simulink model "Hardware_Code"  (R2025b)
settings: Solver=FixedStepAuto  StartTime=0.0  StopTime=30  RelTol=1e-3  EnableMultiTasking=on
InitFcn:
  | battery_init;
  | Full_Charge_Volt=4.2; % unit volts
  | Cutoff_Volt=3; % unit volts
  | Delta=.02;
  | ContactorTime=20;
  | ContactorTimeOut=100;
  | High_TempLim=333;
  | Low_TempLim=253;
  | Sensor_Fault_Treshold=.02;
  | CurrentTimeout=1;
  | Allowed_Delta=.04;
  | Bal_On_Time=30;
  | Bal_Off_Time=5;
  | BalNotAct_Time=10;
values from neighbouring files (symbols this model uses):
  Charge_Rate = 1    [battery_init.m]
  Discharge_Rate = -1    [battery_init.m]
  Fly_Cycle_Current = [ ... (first row only)    [battery_init.m]
undefined symbols (not defined in the file or in its folder): batt, From_Plant_MATLABStruct, SRE
libraries: fl_lib x69, nesl_utility x54, ee_lib x12, batteryecm_lib x12, simulink x6, BatteryCurrentManagement x1
(part 2 of 2)

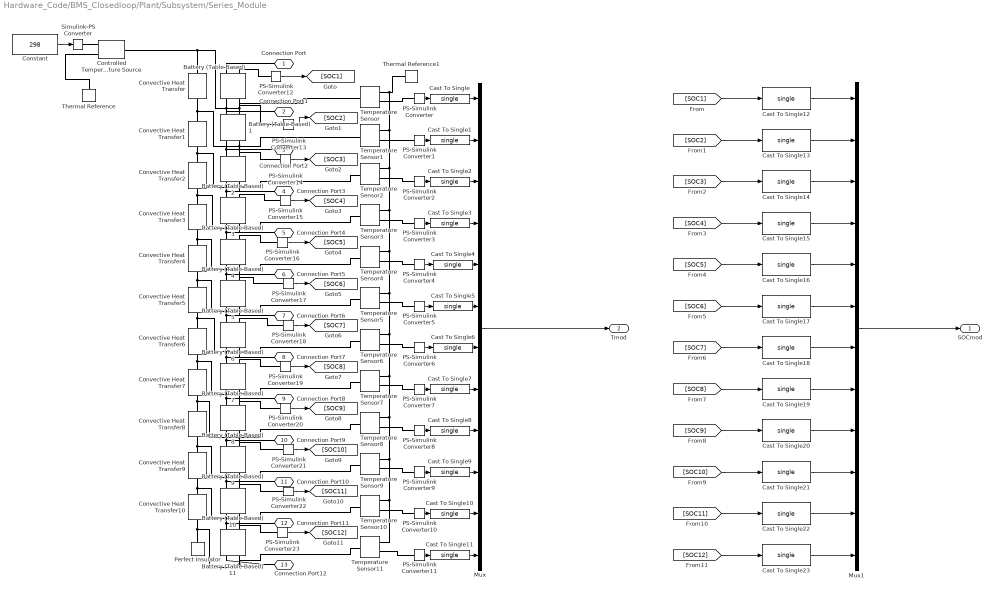
== system Hardware_Code/BMS_Closedloop/Plant/Subsystem/Series_Module ==
  Battery (Table-Based){,1..11} (12 alike) : batteryecm_lib/Battery (Table-Based)  PartSpecification="{\"CollectionId\":\"SimscapeBatteryShared\",\"CollectionVersion\":\"1.0.0\",\"DatasetId\":\"Molicel|INR_21700_P45B|simscape.battery.batteryTableBased\",\"DisplayName\":\"Molicel:INR_21700_P45B\"}"  SOC_vec=[0 0.01 0.02 0.03 0.04 0.05 0.06 0.07 0.08 0.09 0.1 0.11 0.12 0.13 0.14 0.15 0.16 0.17 0.18 0.19 0.2 0.21 0.22 0.23 0.24 0.25 0.26 0.27 0.28 0.29 0.3 0.31 0.32 0.33 0.34 0.35 0.36 0.37 0.38 0.39 0.4 0.41 0.42 0.43 0.44 0.45 0.46 0.47 0.48 0.49 0.5 0.51 0.52 0.53 0.54 0.55 0.56 0.57 0.58 0.59 0.6 0.61 0.62 0.63 0.64 0.65 0.66 0.67 0.68 0.69 0.7 0.71 0.72 0.73 0.74 0.75 0.76 0.77 0.78 0.79 0.8 0.81 0.82 0.83 0.84 0.85 0.86 0.87 0.88 0.89 0.9 0.91 0.92 0.93 0.94 0.95 0.96 0.97 0.98 0.99 1] % Datasheet derived  T_dependence=simscape.enum.tablebattery.temperature_dependence.yes  prm_dir=simscape.enum.tablebattery.prm_dir.noCurrentDirectionality  T_vec=[233.15 243.15 253.15 273.15 296.15 318.15 333.15] K  V0_mat=[3.17242 3.17242 3.17242 3.17242 3.17242 3.17242 3.17242;3.18272 3.18272 3.18272 3.18272 3.18272 3.18272 3.18272;3.19302 3.19302 3.19302 3.19302 3.19302 3.19302 3.19302;3.20331 3.20331 3.20331 3.20331 3.20331 3.20331 3.20331;3.21361 3.21361 3.21361 3.21361 3.21361 3.21361 3.21361;3.22391 3.22391 3.22391 3.22391 3.22391 3.22391 3.22391;3.23421 3.23421 3.23421 3.23421 3.23421 3.23421 3.23421;3.24451 3.24451 3.24451 3.24451 3.24451 3.24451 3.24451;3.25481 3.25481 3.25481 3.25481 3.25481 3.25481 3.25481;3.2651 3.2651 3.2651 3.2651 3.2651 3.2651 3.2651;3.2754 3.2754 3.2754 3.2754 3.2754 3.2754 3.2754;3.2857 3.2857 3.2857 3.2857 3.2857 3.2857 3.2857;3.296 3.296 3.296 3.296 3.296 3.296 3.296;3.3063 3.3063 3.3063 3.3063 3.3063 3.3063 3.3063;3.31659 3.31659 3.31659 3.31659 3.31659 3.31659 3.31659;3.32689 3.32689 3.32689 3.32689 3.32689 3.32689 3.32689;3.33719 3.33719 3.33719 3.33719 3.33719 3.33719 3.33719;3.34749 3.34749 3.34749 3.34749 3.34749 3.34749 3.34749;3.35779 3.35779 3.35779 3.35779 3.35779 3.35779 3.35779;3.36809 3.36809 3.36809 3.36809 3.36809 3.36809 3.36809;3.37838 3.37838 3.37838 3.37838 3.37838 3.37838 3.37838;3.38868 3.38868 3.38868 3.38868 3.38868 3.38868 3.38868;3.39898 3.39898 3.39898 3.39898 3.39898 3.39898 3.39898;3.40928 3.40928 3.40928 3.40928 3.40928 3.40928 3.40928;3.41958 3.41958 3.41958 3.41958 3.41958 3.41958 3.41958;3.42988 3.42988 3.42988 3.42988 3.42988 3.42988 3.42988;3.44017 3.44017 3.44017 3.44017 3.44017 3.44017 3.44017;3.45047 3.45047 3.45047 3.45047 3.45047 3.45047 3.45047;3.46077 3.46077 3.46077 3.46077 3.46077 3.46077 3.46077;3.47107 3.47107 3.47107 3.47107 3.47107 3.47107 3.47107;3.48137 3.48137 3.48137 3.48137 3.48137 3.48137 3.48137;3.49166 3.49166 3.49166 3.49166 3.49166 3.49166 3.49166;3.50196 3.50196 3.50196 3.50196 3.50196 3.50196 3.50196;3.51226 3.51226 3.51226 3.51226 3.51226 3.51226 3.51226;3.52256 3.52256 3.52256 3.52256 3.52256 3.52256 3.52256;3.53286 3.53286 3.53286 3.53286 3.53286 3.53286 3.53286;3.54316 3.54316 3.54316 3.54316 3.54316 3.54316 3.54316;3.55345 3.55345 3.55345 3.55345 3.55345 3.55345 3.55345;3.56375 3.56375 3.56375 3.56375 3.56375 3.56375 3.56375;3.57405 3.57405 3.57405 3.57405 3.57405 3.57405 3.57405;3.58435 3.58435 3.58435 3.58435 3.58435 3.58435 3.58435;3.59465 3.59465 3.59465 3.59465 3.59465 3.59465 3.59465;3.60495 3.60495 3.60495 3.60495 3.60495 3.60495 3.60495;3.61524 3.61524 3.61524 3.61524 3.61524 3.61524 3.61524;3.62554 3.62554 3.62554 3.62554 3.62554 3.62554 3.62554;3.63584 3.63584 3.63584 3.63584 3.63584 3.63584 3.63584;3.64614 3.64614 3.64614 3.64614 3.64614 3.64614 3.64614;3.65644 3.65644 3.65644 3.65644 3.65644 3.65644 3.65644;3.66673 3.66673 3.66673 3.66673 3.66673 3.66673 3.66673;3.67703 3.67703 3.67703 3.67703 3.67703 3.67703 3.67703;3.68733 3.68733 3.68733 3.68733 3.68733 3.68733 3.68733;3.69763 3.69763 3.69763 3.69763 3.69763 3.69763 3.69763;3.71041 3.71041 3.71041 3.71041 3.71041 3.71041 3.71041;3.72113 3.72113 3.72113 3.72113 3.72113 3.72113 3.72113;3.72997 3.72997 3.72997 3.72997 3.72997 3.72997 3.72997;3.73882 3.73882 3.73882 3.73882 3.73882 3.73882 3.73882;3.74912 3.74912 3.74912 3.74912 3.74912 3.74912 3.74912;3.75936 3.75936 3.75936 3.75936 3.75936 3.75936 3.75936;3.76951 3.76951 3.76951 3.76951 3.76951 3.76951 3.76951;3.7791 3.7791 3.7791 3.7791 3.7791 3.7791 3.7791;3.78865 3.78865 3.78865 3.78865 3.78865 3.78865 3.78865;3.79787 3.79787 3.79787 3.79787 3.79787 3.79787 3.79787;3.80709 3.80709 3.80709 3.80709 3.80709 3.80709 3.80709;3.8161 3.8161 3.8161 3.8161 3.8161 3.8161 3.8161;3.82509 3.82509 3.82509 3.82509 3.82509 3.82509 3.82509;3.83409 3.83409 3.83409 3.83409 3.83409 3.83409 3.83409;3.84308 3.84308 3.84308 3.84308 3.84308 3.84308 3.84308;3.85207 3.85207 3.85207 3.85207 3.85207 3.85207 3.85207;3.86107 3.86107 3.86107 3.86107 3.86107 3.86107 3.86107;3.87006 3.87006 3.87006 3.87006 3.87006 3.87006 3.87006;3.87901 3.87901 3.87901 3.87901 3.87901 3.87901 3.87901;3.88831 3.88831 3.88831 3.88831 3.88831 3.88831 3.88831;3.89824 3.89824 ...(+1594 chars)] % Datasheet derived V  V0_vec=[3.17242 3.18272 3.19302 3.20331 3.21361 3.22391 3.23421 3.24451 3.25481 3.2651 3.2754 3.2857 3.296 3.3063 3.31659 3.32689 3.33719 3.34749 3.35779 3.36809 3.37838 3.38868 3.39898 3.40928 3.41958 3.42988 3.44017 3.45047 3.46077 3.47107 3.48137 3.49166 3.50196 3.51226 3.52256 3.53286 3.54316 3.55345 3.56375 3.57405 3.58435 3.59465 3.60495 3.61524 3.62554 3.63584 3.64614 3.65644 3.66673 3.67703 3.68733 3.69763 3.71041 3.72113 3.72997 3.73882 3.74912 3.75936 3.76951 3.7791 3.78865 3.79787 3.80709 3.8161 3.82509 3.83409 3.84308 3.85207 3.86107 3.87006 3.87901 3.88831 3.89824 3.90887 3.91951 3.93012 3.94073 3.95138 3.96184 3.97226 3.98268 3.99311 4.0032 4.01221 4.01944 4.02668 4.03286 4.03874 4.04383 4.0488 4.05377 4.05873 4.06312 4.06753 4.07333 4.08117 4.08904 4.09911 4.11111 4.13802 4.16831] % Datasheet derived V  V_range=[2.25 Inf] % Datasheet derived V  R0_mat=[0.3026 0.35142 0.34349 0.24415 0.02095 0.15874 0.14729;0.2941 0.33555 0.32379 0.22614 0.01921 0.13363 0.12249;0.28559 0.31969 0.30408 0.20813 0.01774 0.10853 0.10276;0.27709 0.30382 0.28438 0.19012 0.0166 0.09423 0.0861;0.26858 0.28796 0.26468 0.17211 0.01557 0.07998 0.0748;0.26008 0.27209 0.24498 0.1541 0.01469 0.07024 0.06679;0.25157 0.25623 0.22527 0.1361 0.01398 0.06387 0.05877;0.24307 0.24036 0.20557 0.11861 0.01338 0.0575 0.05275;0.23456 0.2245 0.18587 0.10674 0.01283 0.05113 0.04899;0.22606 0.20863 0.16617 0.09525 0.01239 0.04679 0.04522;0.21755 0.19277 0.14651 0.08799 0.01196 0.0439 0.04145;0.20905 0.1769 0.13098 0.08073 0.01155 0.04101 0.03817;0.20054 0.16103 0.11905 0.07347 0.01116 0.03813 0.03522;0.19204 0.14769 0.11102 0.06895 0.01079 0.03524 0.03228;0.18353 0.13913 0.10517 0.06499 0.01042 0.03235 0.02934;0.17503 0.13157 0.09933 0.06104 0.01007 0.02946 0.0264;0.16653 0.1271 0.09371 0.05708 0.00974 0.02657 0.02345;0.15804 0.12264 0.09094 0.05312 0.00949 0.02417 0.02125;0.15354 0.11817 0.08816 0.04917 0.00924 0.02286 0.01972;0.14976 0.11385 0.08539 0.04748 0.009 0.02156 0.0182;0.14598 0.11213 0.08261 0.04617 0.00876 0.02025 0.01667;0.14219 0.11042 0.08103 0.04487 0.00855 0.01894 0.01515;0.14033 0.10871 0.08035 0.04356 0.00843 0.01763 0.01363;0.13876 0.10699 0.07967 0.04225 0.00832 0.01632 0.0121;0.13718 0.10528 0.07899 0.04094 0.00826 0.01501 0.01058;0.13561 0.10357 0.07831 0.03964 0.00825 0.0137 0.00906;0.13404 0.10198 0.07763 0.03833 0.00825 0.01239 0.00753;0.13247 0.10119 0.07695 0.03702 0.00826 0.01108 0.0065;0.13096 0.10039 0.07627 0.03624 0.00827 0.00977 0.00633;0.13043 0.0996 0.07559 0.03615 0.00828 0.00846 0.00617;0.1299 0.0988 0.07491 0.03606 0.0083 0.00774 0.006;0.12937 0.09801 0.07423 0.03597 0.00834 0.00779 0.00583;0.12883 0.09721 0.07355 0.03588 0.00838 0.00783 0.00567;0.1283 0.09642 0.07301 0.03579 0.00842 0.00787 0.0055;0.12777 0.09585 0.07296 0.0357 0.00848 0.00792 0.00534;0.12724 0.09584 0.07291 0.03561 0.00855 0.00796 0.00517;0.12675 0.09584 0.07286 0.03552 0.00863 0.00801 0.005;0.12643 0.09583 0.0728 0.03543 0.00871 0.00805 0.00484;0.12611 0.09582 0.07275 0.03534 0.00879 0.00809 0.00467;0.12579 0.09582 0.0727 0.03525 0.00887 0.00814 0.0045;0.12547 0.09581 0.07264 0.03526 0.00895 0.00818 0.00434;0.12514 0.0958 0.07259 0.03537 0.00903 0.00823 0.00405;0.12482 0.09579 0.07254 0.03547 0.00911 0.00804 0.00366;0.1245 0.09579 0.07248 0.03558 0.00918 0.00776 0.00327;0.12418 0.09578 0.07243 0.03568 0.00925 0.00748 0.00287;0.12386 0.09577 0.07231 0.03579 0.00931 0.0072 0.00248;0.12354 0.09576 0.0721 0.03589 0.00938 0.00692 0.00209;0.12322 0.09576 0.07189 0.036 0.00946 0.00664 0.0017;0.12301 0.09575 0.07168 0.03611 0.00953 0.00636 0.00131;0.12309 0.09574 0.07147 0.03621 0.00961 0.00608 0.00092;0.12318 0.09573 0.07125 0.0363 0.00968 0.0058 0.00053;0.12326 0.09573 0.07104 0.03637 0.00976 0.00552 0.00014;0.12389 0.09628 0.07138 0.03699 0.00991 0.00579 0.0003;0.12407 0.09637 0.07126 0.03715 0.01 0.0056 0.0003;0.12383 0.09605 0.07073 0.0369 0.01003 0.00504 0.0003;0.12359 0.09573 0.07019 0.03664 0.01006 0.00503 0.0003;0.12367 0.09573 0.06998 0.03671 0.01013 0.00534 0.00063;0.12375 0.09572 0.06975 0.03677 0.01022 0.00564 0.00094;0.1238 0.09569 0.07006 0.0368 0.0103 0.00593 0.00123;0.12372 0.09554 0.07026 0.03671 0.01037 0.00608 0.00139;0.12364 0.09537 0.07046 0.03661 0.01043 0.00623 0.00155;0.12348 0.09514 0.07058 0.03644 0.01049 0.0063 0.00163;0.12333 0.0949 0.07071 0.03627 0.01055 0.00638 0.00171;0.12312 0.09461 0.07078 0.03605 0.01061 0.00641 0.00175;0.12291 0.09433 0.07085 0.03583 0.01066 0.00643 0.00168;0.12271 0.09404 0.07093 0.03568 0.01072 0.00646 0.00161;0.12275 0.09398 0.071 0.03622 0.01077 0.00646 0.00153;0.12316 0.09449 0.07107 0.03677 0.01082 0.00636 0.00145;0.12357 0.095 0.07115 0.03731 0.01088 0.00625 0.00137;0.12398 0.09551 0.07151 0.03785 0.01093 0.00614 0.00129;0.12438 0.09601 0.07221 0.03839 0.01099 0.00602 0.0012;0.12486 0.09659 0.07299 0.039 0.01105 0.00599 0.00119;0.12548 0.09731 0.07391 ...(+1579 chars)] % Datasheet derived Ohm  R0_vec=[0.02095 0.01921 0.01774 0.0166 0.01557 0.01469 0.01398 0.01338 0.01283 0.01239 0.01196 0.01155 0.01116 0.01079 0.01042 0.01007 0.00974 0.00949 0.00924 0.009 0.00876 0.00855 0.00843 0.00832 0.00826 0.00825 0.00825 0.00826 0.00827 0.00828 0.0083 0.00834 0.00838 0.00842 0.00848 0.00855 0.00863 0.00871 0.00879 0.00887 0.00895 0.00903 0.00911 0.00918 0.00925 0.00931 0.00938 0.00946 0.00953 0.00961 0.00968 0.00976 0.00991 0.01 0.01003 0.01006 0.01013 0.01022 0.0103 0.01037 0.01043 0.01049 0.01055 0.01061 0.01066 0.01072 0.01077 0.01082 0.01088 0.01093 0.01099 0.01105 0.01114 0.01125 0.01136 0.01148 0.01161 0.01175 0.01188 0.01202 0.01215 0.01228 0.01241 0.01253 0.01261 0.01269 0.01275 0.0128 0.01285 0.01289 0.01294 0.01298 0.01296 0.01292 0.01292 0.01288 0.01282 0.0128 0.01232 0.01214 0.00952] % Datasheet derived Ohm  R0_dis_mat=[.0117, .0085, .009; .011, .0085, .009; .0114, .0087, .0092; .0107, .0082, .0088; .0107, .0083, .0091; .0113, .0085, .0089; .0116, .0085, .0089] % Parameter not set Ohm  R0_dis_vec=[.0085, .0085, .0087, .0082, .0083, .0085, .0085] % Parameter not set Ohm  R0_ch_mat=[.0117, .0085, .009; .011, .0085, .009; .0114, .0087, .0092; .0107, .0082, .0088; .0107, .0083, .0091; .0113, .0085, .0089; .0116, .0085, .0089] % Parameter not set Ohm  R0_ch_vec=[.0085, .0085, .0087, .0082, .0083, .0085, .0085] % Parameter not set Ohm  AH=4.493 % Datasheet derived hr*A  prm_leak=simscape.enum.tablebattery.prm_leak.disabled  Rleak_vec=[8000, 7000, 6000] % Parameter not set Ohm  Rleak=7e3 % Parameter not set Ohm  extrapolation_option=simscape.enum.extrapolation.nearest  SOC_port=simscape.enum.tablebattery.enable.yes  prm_dyn=simscape.enum.tablebattery.prm_dyn.off  R1_mat=[.0109, .0029, .0013; .0069, .0024, .0012; .0047, .0026, .0013; .0034, .0016, .001; .0033, .0023, .0014; .0033, .0018, .0011; .0028, .0017, .0011] % Parameter not set Ohm  R1_vec=[.0029, .0024, .0026, .0016, .0023, .0018, .0017] % Parameter not set Ohm  tau1_mat=[20, 36, 39; 31, 45, 39; 109, 105, 61; 36, 29, 26; 59, 77, 67; 40, 33, 29; 25, 39, 33] % Parameter not set s  tau1_vec=[36, 45, 105, 29, 77, 33, 39] % Parameter not set s  R2_mat=[.0109, .0029, .0013; .0069, .0024, .0012; .0047, .0026, .0013; .0034, .0016, .001; .0033, .0023, .0014; .0033, .0018, .0011; .0028, .0017, .0011] % Parameter not set Ohm  R2_vec=[.0029, .0024, .0026, .0016, .0023, .0018, .0017] % Parameter not set Ohm  tau2_mat=[20, 36, 39; 31, 45, 39; 109, 105, 61; 36, 29, 26; 59, 77, 67; 40, 33, 29; 25, 39, 33] % Parameter not set s  tau2_vec=[36, 45, 105, 29, 77, 33, 39] % Parameter not set s  R3_mat=[.0109, .0029, .0013; .0069, .0024, .0012; .0047, .0026, .0013; .0034, .0016, .001; .0033, .0023, .0014; .0033, .0018, .0011; .0028, .0017, .0011] % Parameter not set Ohm  R3_vec=[.0029, .0024, .0026, .0016, .0023, .0018, .0017] % Parameter not set Ohm  tau3_mat=[20, 36, 39; 31, 45, 39; 109, 105, 61; 36, 29, 26; 59, 77, 67; 40, 33, 29; 25, 39, 33] % Parameter not set s  tau3_vec=[36, 45, 105, 29, 77, 33, 39] % Parameter not set s  R4_mat=[.0109, .0029, .0013; .0069, .0024, .0012; .0047, .0026, .0013; .0034, .0016, .001; .0033, .0023, .0014; .0033, .0018, .0011; .0028, .0017, .0011] % Parameter not set Ohm  R4_vec=[.0029, .0024, .0026, .0016, .0023, .0018, .0017] % Parameter not set Ohm  tau4_mat=[20, 36, 39; 31, 45, 39; 109, 105, 61; 36, 29, 26; 59, 77, 67; 40, 33, 29; 25, 39, 33] % Parameter not set s  tau4_vec=[36, 45, 105, 29, 77, 33, 39] % Parameter not set s  R5_mat=[.0109, .0029, .0013; .0069, .0024, .0012; .0047, .0026, .0013; .0034, .0016, .001; .0033, .0023, .0014; .0033, .0018, .0011; .0028, .0017, .0011] % Parameter not set Ohm  R5_vec=[.0029, .0024, .0026, .0016, .0023, .0018, .0017] % Parameter not set Ohm  tau5_mat=[20, 36, 39; 31, 45, 39; 109, 105, 61; 36, 29, 26; 59, 77, 67; 40, 33, 29; 25, 39, 33] % Parameter not set s  tau5_vec=[36, 45, 105, 29, 77, 33, 39] % Parameter not set s  prm_fade=simscape.enum.tablebattery.prm_fade.tableN  N0=100 % Parameter not set  dV0=0 % Parameter not set  dR0=0 % Parameter not set  dAH=0 % Parameter not set  dRleak=0 % Parameter not set  dR1=0 % Parameter not set  dR2=0 % Parameter not set  dR3=0 % Parameter not set  dR4=0 % Parameter not set  dR5=0 % Parameter not set  N0vec=[0 6 11 16 21 26 31 36 41 46 51 56 61 66 71 76 81 86 91 96 101 106 111 116 121 126 131 136 141 146 151 156 161 166 171 176 181 186 191 196 201 206 211 216 221 226 231 236 241 246 251 256 261 266 271 276 281 286 291 296 301 306 311 316 321 326 331 336 341 346 351 356 361 366 371 376 381 386 391 396 401 406 411 416 421 426 431 436 441 446 451 456 461 466 471 476 481 486 491 496] % Datasheet derived  Tfadevec=[298.15, 323.15] % Parameter not set K  dV0vec=[0 -0.0674 -0.1349 -0.2023 -0.2697 -0.3371 -0.4046 -0.472 -0.5394 -0.6069 -0.6828 -0.7561 -0.8245 -0.8929 -0.9613 -1.0297 -1.0981 -1.1664 -1.2348 -1.3032 -1.3773 -1.4186 -1.4598 -1.5011 -1.5424 -1.5836 -1.6249 -1.6652 -1.6999 -1.7345 -1.7691 -1.8038 -1.8384 -1.8731 -1.908 -1.9398 -1.9715 -2.0033 -2.0351 -2.0669 -2.0986 -2.1303 -2.162 -2.1976 -2.2332 -2.2687 -2.2977 -2.3239 -2.3502 -2.3765 -2.4028 -2.4264 -2.4464 -2.4663 -2.4863 -2.5063 -2.5263 -2.5462 -2.5661 -2.5849 -2.6031 -2.6212 -2.6407 -2.6612 -2.6817 -2.7022 -2.7227 -2.7432 -2.7637 -2.7842 -2.8047 -2.8253 -2.8458 -2.8662 -2.8858 -2.9054 -2.9249 -2.9445 -2.9641 -2.9837 -3.0037 -3.0238 -3.0439 -3.064 -3.0841 -3.1042 -3.1267 -3.1499 -3.1731 -3.1989 -3.2248 -3.2508 -3.2781 -3.3053 -3.3326 -3.3598 -3.387 -3.4171 -3.449 -3.4809] % Datasheet derived  dR0vec=[0 0 0 0 0 0 0 0 0 0 0 0 0 0 0 0 0 0 0 0 0 0 0 0 0 0 0 0 0 0 0 0 0 0 0 0 0 0 0 0 0 0 0 0 0 0 0 0 0 0 0 0 0 0 0 0 0 0 0 0 0 0 0 0 0 0 0 0 0 0 0 0 0 0 0 0 0 0 0 0 0 0 0 0 0 0 0 0 0 0 0 0 0 0 0 0 0 0 0 0] % Parameter assumed  dAHvec=[0 -0.093 -0.186 -0.278 -0.371 -0.464 -0.557 -0.649 -0.742 -0.835 -0.94 -1.045 -1.151 -1.257 -1.363 -1.469 -1.575 -1.681 -1.787 -1.893 -2.017 -2.161 -2.304 -2.447 -2.591 -2.734 -2.877 -3.021 -3.164 -3.307 -3.451 -3.594 -3.737 -3.881 -4.032 -4.201 -4.369 -4.538 -4.706 -4.874 -5.043 -5.211 -5.38 -5.569 -5.758 -5.947 -6.135 -6.324 -6.513 -6.702 -6.891 -7.08 -7.269 -7.458 -7.647 -7.836 -8.025 -8.214 -8.403 -8.582 -8.754 -8.927 -9.099 -9.271 -9.443 -9.615 -9.787 -9.96 -10.132 -10.304 -10.476 -10.648 -10.82 -10.992 -11.156 -11.32 -11.485 -11.649 -11.814 -11.978 -12.143 -12.307 -12.471 -12.636 -12.8 -12.965 -13.129 -13.293 -13.458 -13.641 -13.825 -14.008 -14.192 -14.376 -14.56 -14.743 -14.927 -15.111 -15.295 -15.478] % Datasheet derived  dRleakvec=[0, 0, 0, 0] % Parameter not set  dR1vec=[0, 0, 0, 0] % Parameter not set  dR2vec=[0, 0, 0, 0] % Parameter not set  dR3vec=[0, 0, 0, 0] % Parameter not set  dR4vec=[0, 0, 0, 0] % Parameter not set  dR5vec=[0, 0, 0, 0] % Parameter not set  dV0mat=[0, 0; 0, 0; 0, 0; 0, 0] % Parameter not set  dR0mat=[0, 0; 0, 0; 0, 0; 0, 0] % Parameter not set  dAHmat=[0, 0; 0, 0; 0, 0; 0, 0] % Parameter not set  dRleakmat=[0, 0; 0, 0; 0, 0; 0, 0] % Parameter not set  dR1mat=[0, 0; 0, 0; 0, 0; 0, 0] % Parameter not set  dR2mat=[0, 0; 0, 0; 0, 0; 0, 0] % Parameter not set  dR3mat=[0, 0; 0, 0; 0, 0; 0, 0] % Parameter not set  dR4mat=[0, 0; 0, 0; 0, 0; 0, 0] % Parameter not set  dR5mat=[0, 0; 0, 0; 0, 0; 0, 0] % Parameter not set  prm_age_modeling=simscape.enum.tablebattery.prm_age_modeling.equation  storage_dt_age_vec=[0] % Parameter not set d  storage_T_age_vec=[273] % Parameter not set K  prm_age_OCV=simscape.enum.tablebattery.prm_age_OCV.OCV  OCV_age=0.9 % Parameter not set  SOC_age=0.6 % Parameter not set  prm_age_resistance=simscape.enum.tablebattery.prm_age.disabled  OCV_scaling_age_resistance=2.2134e6 % Parameter not set  OCV_offset_age_resistance=1.632e6 % Parameter not set  temp_exp_age_resistance=0.515833569 % Parameter not set V  t_exp_age_resistance=0.75 % Parameter not set  T_age_vec_resistance=[273.15, 298.15, 323.15] % Parameter not set K  dt_age_vec_resistance=[0, 90, 180, 270] % Parameter not set d  dR0_age_vec=[0, 0, 0] % Parameter not set  t_meas_dR0_age=100 % Parameter not set d  dR0_age_mat=[0, 0, 0; 0, 0, 0; 0, 0, 0; 0, 0, 0] % Parameter not set  prm_age_capacity=simscape.enum.tablebattery.prm_age.disabled  OCV_scaling_age_capacity=1.5097e07 % Parameter not set  OCV_offset_age_capacity=8.3625e06 % Parameter not set  temp_exp_age_capacity=0.6011 % Parameter not set V  t_exp_age_capacity=0.75 % Parameter not set  T_age_vec_capacity=[273.15, 298.15, 323.15] % Parameter not set K  dt_age_vec_capacity=[0, 90, 180, 270] % Parameter not set d  dAH_age_vec=[0, 0, 0] % Parameter not set  t_meas_dAH_age=100 % Parameter not set d  dAH_age_mat=[0, 0, 0; 0, 0, 0; 0, 0, 0; 0, 0, 0] % Parameter not set  thermal_port=simscape.enum.thermaleffects.model  temperature=298.15 % Parameter not set K  thermal_mass=63 % Parameter assumed J/K  i_specify=off  i_priority=None  i=0 A  i_nominal_specify=off  i_nominal_value=1  i_nominal_unit=A  v_specify=off  v_priority=None  v=0 V  v_nominal_specify=off  v_nominal_value=1  v_nominal_unit=V  stateOfCharge_specify=on  stateOfCharge_priority=High  stateOfCharge=1  stateOfCharge_nominal_specify=off  stateOfCharge_nominal_value=1  stateOfCharge_nominal_unit=1  num_cycles_specify=off  num_cycles_priority=High  num_cycles=0  num_cycles_nominal_specify=off  num_cycles_nominal_value=1  num_cycles_nominal_unit=1  cell_temperature_specify=on  cell_temperature_priority=High  cell_temperature=298.15 K  cell_temperature_nominal_specify=off  cell_temperature_nominal_value=1  cell_temperature_nominal_unit=K
      settings: AttributesFormatString=Molicel:INR_21700_P45B
      settings: LibrarySourceBlock=|
      | batt_lib/Cells/Battery
      | (Table-Based)
  Cast To Single{,1..23} (24 alike) : DataTypeConversion  OutDataTypeStr=single  SaturateOnIntegerOverflow=off  RndMeth=Floor
  Constant : Constant  Value=298
  Controlled Temperature Source : fl_lib/Thermal/Thermal Sources/Controlled Temperature Source
  Convective Heat Transfer{,1..10} (11 alike) : fl_lib/Thermal/Thermal Elements/Convective Heat Transfer  thermal_type=foundation.enum.constant_variable.constant  area=1e-4 m^2  heat_tr_coeff=20 W/(K*m^2)  min_heat_tr_coeff=1e-3 W/(K*m^2)  T_specify=off  T_priority=None  T=0 K  T_nominal_specify=off  T_nominal_value=1  T_nominal_unit=K  Q_specify=off  Q_priority=None  Q=0 W  Q_nominal_specify=off  Q_nominal_value=1  Q_nominal_unit=W
  Mux : Mux  Inputs=12
  Mux1 : Mux  Inputs=12
  PS-Simulink Converter{,1..23} (24 alike) : nesl_utility/PS-Simulink Converter  PhysicalDomain=network_engine_domain  SubClassName=ps_output  LeftPortType=input  RightPortType=output  PseudoPeriodic=off  Frequencies=[]  VectorFormat=inherit  Unit=inherit  AffineConversion=off
  Perfect Insulator : fl_lib/Thermal/Thermal Elements/Perfect Insulator  T_specify=off  T_priority=None  T=293.15 K  T_nominal_specify=off  T_nominal_value=1  T_nominal_unit=K
  Simulink-PS Converter : nesl_utility/Simulink-PS Converter  PhysicalDomain=network_engine_domain  SubClassName=ps_input  LeftPortType=input  RightPortType=output  PseudoPeriodic=off  Frequencies=[]  NoiseDistribution=none  NoiseParameters=[]  Unit=1  AffineConversion=off  FilteringAndDerivatives=provide  SimscapeFilterOrder=1  InputFilterTimeConstant=0.001  UdotUserProvided=0
  Temperature Sensor{,1..11} (12 alike) : fl_lib/Thermal/Thermal Sensors/Temperature Sensor  temperature_measure=foundation.enum.MeasurementReference.difference
  Thermal Reference : fl_lib/Thermal/Thermal Elements/Thermal Reference
  Thermal Reference1 : fl_lib/Thermal/Thermal Elements/Thermal Reference
  Connection Port : PMIOPort  Side=Left
  Connection Port1 : PMIOPort  Port=2  Side=Left
  Connection Port2 : PMIOPort  Port=3  Side=Left
  Connection Port3 : PMIOPort  Port=4  Side=Left
  Connection Port4 : PMIOPort  Port=5  Side=Left
  Connection Port5 : PMIOPort  Port=6  Side=Left
  Connection Port6 : PMIOPort  Port=7  Side=Left
  Connection Port7 : PMIOPort  Port=8  Side=Left
  Connection Port8 : PMIOPort  Port=9  Side=Left
  Connection Port9 : PMIOPort  Port=10  Side=Left
  Connection Port10 : PMIOPort  Port=11  Side=Left
  Connection Port11 : PMIOPort  Port=12  Side=Left
  Connection Port12 : PMIOPort  Port=13  Side=Left
  SOCmod : Outport
  Tmod : Outport  Port=2
  wires:
  Constant/1 -> Simulink-PS Converter/1
  PS-Simulink Converter12/1 -> [SOC1]
  PS-Simulink Converter13/1 -> [SOC2]
  PS-Simulink Converter14/1 -> [SOC3]
  PS-Simulink Converter15/1 -> [SOC4]
  PS-Simulink Converter16/1 -> [SOC5]
  PS-Simulink Converter17/1 -> [SOC6]
  PS-Simulink Converter18/1 -> [SOC7]
  PS-Simulink Converter19/1 -> [SOC8]
  PS-Simulink Converter20/1 -> [SOC9]
  PS-Simulink Converter21/1 -> [SOC10]
  PS-Simulink Converter22/1 -> [SOC11]
  PS-Simulink Converter23/1 -> [SOC12]
  [SOC1] -> Cast To Single12/1
  [SOC2] -> Cast To Single13/1
  [SOC3] -> Cast To Single14/1
  [SOC4] -> Cast To Single15/1
  [SOC5] -> Cast To Single16/1
  [SOC6] -> Cast To Single17/1
  [SOC7] -> Cast To Single18/1
  [SOC8] -> Cast To Single19/1
  [SOC9] -> Cast To Single20/1
  [SOC10] -> Cast To Single21/1
  [SOC11] -> Cast To Single22/1
  [SOC12] -> Cast To Single23/1
  Cast To Single/1 -> Mux/1
  PS-Simulink Converter/1 -> Cast To Single/1
  Cast To Single1/1 -> Mux/2
  PS-Simulink Converter1/1 -> Cast To Single1/1
  Cast To Single2/1 -> Mux/3
  PS-Simulink Converter2/1 -> Cast To Single2/1
  PS-Simulink Converter3/1 -> Cast To Single3/1
  Cast To Single3/1 -> Mux/4
  PS-Simulink Converter4/1 -> Cast To Single4/1
  Cast To Single4/1 -> Mux/5
  PS-Simulink Converter5/1 -> Cast To Single5/1
  Cast To Single5/1 -> Mux/6
  Cast To Single6/1 -> Mux/7
  PS-Simulink Converter6/1 -> Cast To Single6/1
  PS-Simulink Converter7/1 -> Cast To Single7/1
  Cast To Single7/1 -> Mux/8
  PS-Simulink Converter8/1 -> Cast To Single8/1
  Cast To Single8/1 -> Mux/9
  PS-Simulink Converter9/1 -> Cast To Single9/1
  Cast To Single9/1 -> Mux/10
  PS-Simulink Converter10/1 -> Cast To Single10/1
  Cast To Single10/1 -> Mux/11
  PS-Simulink Converter11/1 -> Cast To Single11/1
  Cast To Single11/1 -> Mux/12
  Mux/1 -> Tmod/1
  Mux1/1 -> SOCmod/1
  Cast To Single12/1 -> Mux1/1
  Cast To Single13/1 -> Mux1/2
  Cast To Single14/1 -> Mux1/3
  Cast To Single15/1 -> Mux1/4
  Cast To Single16/1 -> Mux1/5
  Cast To Single17/1 -> Mux1/6
  Cast To Single18/1 -> Mux1/7
  Cast To Single19/1 -> Mux1/8
  Cast To Single20/1 -> Mux1/9
  Cast To Single21/1 -> Mux1/10
  Cast To Single22/1 -> Mux1/11
  Cast To Single23/1 -> Mux1/12
  connections:
  Battery (Table-Based)1/LConn1 -- Connection Port1/RConn1 -- Battery (Table-Based)/RConn1
  Battery (Table-Based)2/LConn1 -- Connection Port2/RConn1 -- Battery (Table-Based)1/RConn1
  Battery (Table-Based)8/LConn1 -- Connection Port8/RConn1 -- Battery (Table-Based)7/RConn1
  Battery (Table-Based)3/LConn1 -- Connection Port3/RConn1 -- Battery (Table-Based)2/RConn1
  Battery (Table-Based)5/LConn1 -- Connection Port5/RConn1 -- Battery (Table-Based)4/RConn1
  Convective Heat Transfer3/LConn1 -- Temperature Sensor3/LConn1 -- Battery (Table-Based)3/RConn2 -- Convective Heat Transfer2/RConn1
  Battery (Table-Based)8/RConn2 -- Temperature Sensor8/LConn1 -- Convective Heat Transfer7/RConn1 -- Convective Heat Transfer8/LConn1
  Convective Heat Transfer10/LConn1 -- Temperature Sensor10/LConn1 -- Battery (Table-Based)10/RConn2 -- Convective Heat Transfer9/RConn1
  Battery (Table-Based)9/LConn1 -- Connection Port9/RConn1 -- Battery (Table-Based)8/RConn1
  Battery (Table-Based)/RConn2 -- Temperature Sensor/LConn1 -- Convective Heat Transfer/LConn1 -- Controlled Temperature Source/LConn1
  Battery (Table-Based)10/LConn1 -- Connection Port10/RConn1 -- Battery (Table-Based)9/RConn1
  Convective Heat Transfer7/LConn1 -- Temperature Sensor7/LConn1 -- Battery (Table-Based)7/RConn2 -- Convective Heat Transfer6/RConn1
  Convective Heat Transfer10/RConn1 -- Temperature Sensor11/LConn1 -- Battery (Table-Based)11/RConn2 -- Perfect Insulator/LConn1
  Convective Heat Transfer1/LConn1 -- Temperature Sensor1/LConn1 -- Battery (Table-Based)1/RConn2 -- Convective Heat Transfer/RConn1
  Convective Heat Transfer4/LConn1 -- Temperature Sensor4/LConn1 -- Battery (Table-Based)4/RConn2 -- Convective Heat Transfer3/RConn1
  Battery (Table-Based)6/LConn1 -- Connection Port6/RConn1 -- Battery (Table-Based)5/RConn1
  Battery (Table-Based)4/LConn1 -- Connection Port4/RConn1 -- Battery (Table-Based)3/RConn1
  Battery (Table-Based)7/LConn1 -- Connection Port7/RConn1 -- Battery (Table-Based)6/RConn1
  Convective Heat Transfer6/LConn1 -- Temperature Sensor6/LConn1 -- Battery (Table-Based)6/RConn2 -- Convective Heat Transfer5/RConn1
  Battery (Table-Based)11/LConn1 -- Connection Port11/RConn1 -- Battery (Table-Based)10/RConn1
  Thermal Reference/LConn1 -- Controlled Temperature Source/RConn2
  Controlled Temperature Source/RConn1 -- Simulink-PS Converter/RConn1
  Convective Heat Transfer9/LConn1 -- Temperature Sensor9/LConn1 -- Battery (Table-Based)9/RConn2 -- Convective Heat Transfer8/RConn1
  Convective Heat Transfer5/LConn1 -- Temperature Sensor5/LConn1 -- Battery (Table-Based)5/RConn2 -- Convective Heat Transfer4/RConn1
  Battery (Table-Based)/LConn1 -- Connection Port/RConn1
  Convective Heat Transfer2/LConn1 -- Temperature Sensor2/LConn1 -- Battery (Table-Based)2/RConn2 -- Convective Heat Transfer1/RConn1
  Connection Port12/RConn1 -- Battery (Table-Based)11/RConn1
  Thermal Reference1/LConn1 -- Temperature Sensor11/RConn1 -- Temperature Sensor10/RConn1 -- Temperature Sensor9/RConn1 -- Temperature Sensor8/RConn1 -- Temperature Sensor7/RConn1 -- Temperature Sensor6/RConn1 -- Temperature Sensor5/RConn1 -- Temperature Sensor4/RConn1 -- Temperature Sensor3/RConn1 -- Temperature Sensor2/RConn1 -- Temperature Sensor1/RConn1 -- Temperature Sensor/RConn1
  Temperature Sensor/RConn2 -- PS-Simulink Converter/LConn1
  PS-Simulink Converter1/LConn1 -- Temperature Sensor1/RConn2
  Temperature Sensor11/RConn2 -- PS-Simulink Converter11/LConn1
  Temperature Sensor10/RConn2 -- PS-Simulink Converter10/LConn1
  Temperature Sensor9/RConn2 -- PS-Simulink Converter9/LConn1
  Temperature Sensor8/RConn2 -- PS-Simulink Converter8/LConn1
  Temperature Sensor7/RConn2 -- PS-Simulink Converter7/LConn1
  Temperature Sensor6/RConn2 -- PS-Simulink Converter6/LConn1
  Temperature Sensor5/RConn2 -- PS-Simulink Converter5/LConn1
  Temperature Sensor4/RConn2 -- PS-Simulink Converter4/LConn1
  Temperature Sensor3/RConn2 -- PS-Simulink Converter3/LConn1
  Temperature Sensor2/RConn2 -- PS-Simulink Converter2/LConn1
  PS-Simulink Converter12/LConn1 -- Battery (Table-Based)/LConn2
  Battery (Table-Based)1/LConn2 -- PS-Simulink Converter13/LConn1
  Battery (Table-Based)2/LConn2 -- PS-Simulink Converter14/LConn1
  PS-Simulink Converter15/LConn1 -- Battery (Table-Based)3/LConn2
  PS-Simulink Converter16/LConn1 -- Battery (Table-Based)4/LConn2
  Battery (Table-Based)5/LConn2 -- PS-Simulink Converter17/LConn1
  PS-Simulink Converter18/LConn1 -- Battery (Table-Based)6/LConn2
  PS-Simulink Converter19/LConn1 -- Battery (Table-Based)7/LConn2
  Battery (Table-Based)8/LConn2 -- PS-Simulink Converter20/LConn1
  Battery (Table-Based)9/LConn2 -- PS-Simulink Converter21/LConn1
  Battery (Table-Based)10/LConn2 -- PS-Simulink Converter22/LConn1
  Battery (Table-Based)11/LConn2 -- PS-Simulink Converter23/LConn1

== stateflow chart Hardware_Code/Test Sequence ==
  state Flying
    State_Required=SRE.Flying
  state Standby
    State_Required=SRE.Standby
  state Charging
    State_Required=SRE.Charge
  (default) -> Flying
  Flying -> Standby : [
      | after(10, sec)
      | ]
  Standby -> Charging : [
      | after(5, sec)
      | ]
  data: State_Required output Enum: SRE

== stateflow chart Hardware_Code/BMS_Closedloop/BMS_Control/Subsystem1/Chart ==
  state Balancing_Off
    en:
    Bal_Cmd(:,:)= false;
    en, du:
    DeltaCellVolt=Max_Voltage-Min_Voltage;
  state Balancing_On
    en, du:
    DeltaCellVolt=Max_Voltage-Min_Voltage;
    state Balance_Active
      en, du:
      Bal_Cmd=((Vmod-Min_Voltage)> Allowed_Delta/2)';
      flgBalCompl=all(~Bal_Cmd);
    state Balance_Not_Active
    (default) -> Balance_Active
    Balance_Not_Active -> Balance_Active [order 1] : [after(BalNotAct_Time, sec) &&...
        |  DeltaCellVolt> Allowed_Delta]
    Balance_Active -> Balance_Not_Active : [flgBalCompl]
  (default) -> Balancing_Off : {flgBalCompl}
  Balancing_Off -> Balancing_On : [flgBalCompl &&...
      | BMS_State_Out~=BMS_State.Flying &&...
      | after(Bal_Off_Time, sec) &&...
      | DeltaCellVolt> Allowed_Delta]
  Balancing_On -> Balancing_Off : [BMS_State_Out==BMS_State.Flying]
  Balance_Not_Active -> Balancing_Off [order 2] : [after(Bal_On_Time, sec)]
  data: BMS_State_Out input; Min_Voltage input single; Max_Voltage input single; Bal_Cmd output boolean; flgBalCompl local boolean =false; Allowed_Delta parameter single; DeltaCellVolt local single; Bal_On_Time parameter single; Bal_Off_Time parameter single; BalNotAct_Time parameter single; Vmod input single

== matlab function Hardware_Code/BMS_Closedloop/BMS_Control/SOC estimator/MATLAB Function ==
  data: soc input; soc0 output
function soc0 = get_initial_soc(soc)

persistent first_value

if isempty(first_value)
    first_value = soc;
end

soc0 = first_value;

== stateflow chart Hardware_Code/BMS_Closedloop/BMS_Control/Subsystem/BMS_States ==
  state Normal_State [parallel]
    settings: executionOrder=2
    state Standby
      en:
      BMS_State_Out= BMS_State.Standby
    state Charging
      en:
      BMS_State_Out= BMS_State.Charge
    state Flying
      en:
      BMS_State_Out= BMS_State.Flying
    state Fault
      en,du:
      BMS_State_Out= BMS_State.Fault
    (default) -> Standby
    Standby -> Charging [order 2] : [State_Required==SRE.Charge ]
    Standby -> (junction 51) [order 3] : [FaultPresent]
    (junction 51) -> (junction 52)
    Charging -> Standby [order 1] : [(State_Required~=SRE.Charge)...
        | || (State_Required==SRE.Standby) ]
    Standby -> Flying [order 1] : [State_Required== SRE.Flying]
    Flying -> Standby [order 1] : [(State_Required~=SRE.Flying) ||...
        | (State_Required==SRE.Standby) ]
    (junction 43) -> Charging
    Charging -> (junction 41) [order 2]
    Charging -> Fault [order 3] : [FaultPresent]
    Flying -> (junction 43) [order 2] : [State_Required==SRE.Charge]
    (junction 41) -> Flying : [State_Required== SRE.Flying]
    Flying -> Fault [order 3] : [FaultPresent]
    (junction 52) -> Fault
  state Fault_Monitoring [parallel]
    settings: executionOrder=1
    state Monitor_CurrentLim [parallel]
      settings: executionOrder=1
      state No_CurrentLim_Fault
      state Wait
      state OC_Fault
        en:
        FaultPresent=true;
        Fault_out.OC=true;
      (default) -> No_CurrentLim_Fault : {FaultPresent=false;
          |  Fault_out.OC=false;}
      No_CurrentLim_Fault -> Wait : [(Pack_Current< Current_Limits.Discharge_Current_Limit) || ...
          | (Pack_Current> Current_Limits.Charge_Current_Limit)]
      Wait -> No_CurrentLim_Fault [order 2] : [(Pack_Current >= Current_Limits.Discharge_Current_Limit) && ...
          | (Pack_Current <= Current_Limits.Charge_Current_Limit)]
      Wait -> OC_Fault [order 1] : [after(CurrentTimeout, sec)]
    state Monitor_CellVolt [parallel]
      settings: executionOrder=2
      state No_OV_UV
        en,du:
        Volt_sum=sum(Vmod);
        Delta=abs(Pack_Volt-Volt_sum);
      state OV_Fault
        en:
        FaultPresent=true;
        Fault_out.OV=true;
      state Sensor_Fault
        en:
        FaultPresent=true;
        Fault_out.VoltSensor=true;
      state UV_Fault
        en:
        FaultPresent=true;
        Fault_out.UV=true;
      (default) -> No_OV_UV : {FaultPresent=false;
          | Fault_out.VoltSensor=false;
          | Fault_out.UV=false;
          | Fault_out.OV=false;}
      No_OV_UV -> OV_Fault [order 3] : [Max_Voltage>=Full_Charge_Volt]
      No_OV_UV -> (junction 89) [order 2] : [Min_Voltage <= Cutoff_Volt]
      (junction 89) -> UV_Fault
      (junction 173) -> No_OV_UV : [[Min_Voltage > Cutoff_Volt]]
      UV_Fault -> (junction 173)
      No_OV_UV -> Sensor_Fault [order 1] : [Delta>=single(Sensor_Fault_Treshold)]
    state Monitor_CellTemp [parallel]
      settings: executionOrder=3
      state OT_Fault
        en:
        FaultPresent=true;
        Fault_out.OT=true;
      state No_OT_UT
        en, du:
        MaxCellTemp=max(Tmod);
        MinCellTemp=min(Tmod);
        FaultPresent=false;
        Fault_out.OT=false;
        Fault_out.UT=false;
      state UT_Fault
        en:
        FaultPresent=true;
        Fault_out.UT=true;
      No_OT_UT -> OT_Fault [order 2] : [MaxCellTemp>=High_TempLim]
      (default) -> No_OT_UT : {FaultPresent=false;
          | Fault_out.OT=false;
          | Fault_out.UT=false;}
      No_OT_UT -> UT_Fault [order 1] : [MinCellTemp<=Low_TempLim]
  data: Current_Limits input Bus: Current_Limits; Vmod input single; Tmod input single; Pack_Current input single; Pack_Volt input single size=1; State_Required input Enum: SRE; Fault_out output Bus: Fault_out; Max_Voltage input single; Min_Voltage input single; Low_TempLim parameter single; High_TempLim parameter single; Cutoff_Volt parameter single; Full_Charge_Volt parameter single; MaxCellTemp local single; MinCellTemp local single; Volt_sum local single; Delta local single; Sensor_Fault_Treshold parameter double; FaultPresent local boolean; BMS_State_Out output; CurrentTimeout parameter
